simulink model "generate_cartesian_pose_motion"  (R2023a)
settings: Solver=FixedStepDiscrete  StartTime=0.0  StopTime=inf  FixedStep=0.001  RelTol=1e-3  EnableMultiTasking=on
PreLoadFcn:
  | frs = FrankaRobotSettings;
libraries: franka_simulink_library x4
settings Model: SimulationMode=external  ExtModeTrigDuration=10000  Creator=vasi_ko  LastModifiedBy=kvasios
settings SolverCC: AlgebraicLoopSolver=TrustRegion
settings DataIOCC: LimitDataPoints=on  SaveFormat=Array  ReturnWorkspaceOutputs=off
settings OptimizationCC: DefaultParameterBehavior=Inlined  EnhancedBackFolding=on  PassReuseOutputArgsThreshold=0  OptimizeBlockOrder=speed  DifferentSizesBufferReuse=on  OptimizationCustomize=off
settings DebuggingCC: SolverPrmCheckMsg=warning  ParameterTunabilityLossMsg=error  UnconnectedInputMsg=warning  UnconnectedOutputMsg=warning  UnconnectedLineMsg=warning  SFUnexpectedBacktrackingDiag=warning  SFNoUnconditionalDefaultTransitionDiag=warning  SFExecutionAtInitializationDiag=none  ArithmeticOperatorsInVariantConditions=warning
settings ModelReferenceCC: EnableRefExpFcnMdlSchedulingChecks=on  PropagateSignalLabelsOutOfModel=off
settings SFSimCC: SimUseLocalCustomCode=off  MATLABDynamicMemAlloc=off  CustomCodeUndefinedFunction=UseInterfaceOnly  SimTargetLang=C++
settings RTWCC: RTWVerbose=off  RTWUseLocalCustomCode=off  BuildConfiguration=Faster Runs  TargetLang=C++  DLArmComputeVersion=19.05
settings CodeAppCC: ForceParamTrailComments=on  OperatorAnnotations=on
settings ConfigComp: CovMetricSettings=dw  CovSaveCumulativeToWorkspaceVar=on  CovSaveSingleToWorkspaceVar=on  CovExternalEMLEnable=off  CovSFcnEnable=off

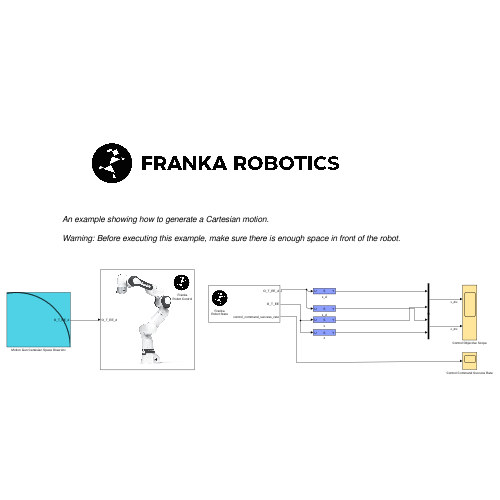
[thumbnail: Simulink's stored preview of the top-level diagram]
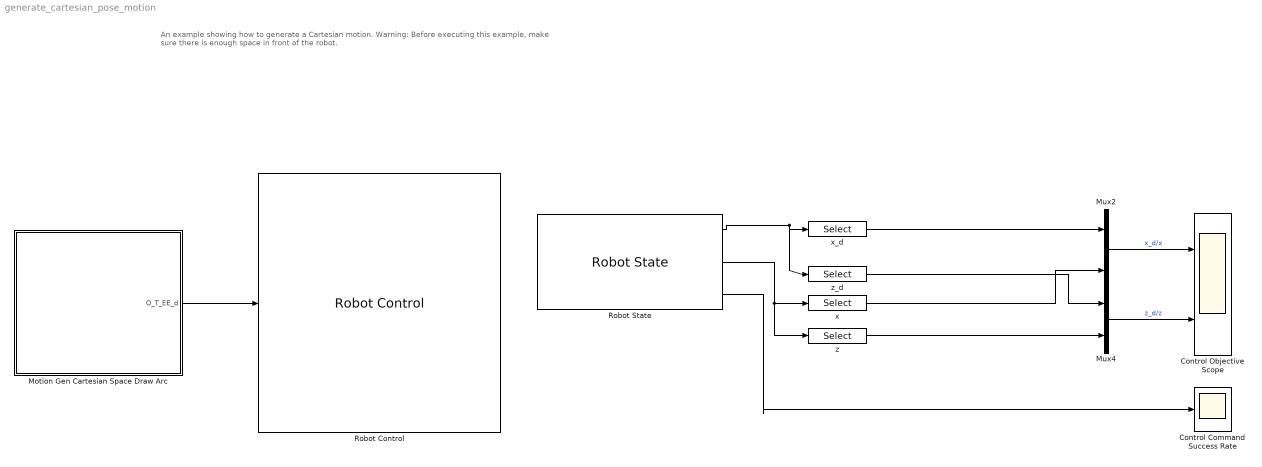
== system generate_cartesian_pose_motion ==
  note: An example showing how to generate a Cartesian motion.
      |
      | Warning: Before executing this example, make sure there is enough space in front of the robot.
  Control Command Success Rate : Scope
  Control Objective Scope : Scope  NumInputPorts=2
  Motion Gen Cartesian Space Draw Arc : Subsystem
      mask Display:
      | pos = get_param(gcb, 'Position');
      | width = pos(3) - pos(1);
      | x = [0:width];
      | y = sin(x/180*pi);
      | % Parameters 'm' and 'b' must be defined in 'Parameters & Dialog' pane.
      | plot(cos(x/180*pi*0.5), sin(x/180*pi*0.5));
      | 
      | port_label('output',1,'O_T_EE_d');
  Mux2 : Mux  Inputs=2
  Mux4 : Mux  Inputs=2
  Robot Control : franka_simulink_library/Robot Control  robot_ip=frs.robot_ip  gripper_selection=None  control_mode=Cartesian Pose - Internal Controller Mode  controller_choice=Joint Impedance Controller  joint_impedance=frs.joint_impedance_stiffness  cartesian_impedance=[3000, 3000, 3000, 300, 300, 300]  rate_limiter=on  cuttoff_frequency=frs.cutoff_frequency  elbow_control=off  collision_thresholds=frs.collision_thresholds.getAs1DArray  load_inertia=frs.load_inertia.getAs1DArray  NE_T_EE=frs.NE_T_EE(:)  EE_T_K=frs.EE_T_K(:)  init_joint_configuration_req=on  init_joint_configuration=frs.home_configuration
      settings: SourceProductName=Franka Robotics Simulink Support Package
  Robot State : franka_simulink_library/Robot State  robot_ip=frs.robot_ip  signals_requested='O_T_EE_d O_T_EE control_command_success_rate'
      settings: SourceProductName=Franka Robotics Simulink Support Package
  x : Selector  InputPortWidth=16  IndexOptions=Index vector (dialog)  Indices=13  OutputSizes=1
  x_d : Selector  InputPortWidth=16  IndexOptions=Index vector (dialog)  Indices=13  OutputSizes=1
  z : Selector  InputPortWidth=16  IndexOptions=Index vector (dialog)  Indices=15  OutputSizes=1
  z_d : Selector  InputPortWidth=16  IndexOptions=Index vector (dialog)  Indices=15  OutputSizes=1
  wires:
  x/1 -> Mux2/2
  z/1 -> Mux4/2
  Mux2/1 -> Control Objective Scope/1  "x_d/x"
  Mux4/1 -> Control Objective Scope/2  "z_d/z"
  Robot State/1 -> z_d/1, x_d/1
  x_d/1 -> Mux2/1
  Motion Gen Cartesian Space Draw Arc/1(O_T_EE_d) -> Robot Control/1
  z_d/1 -> Mux4/1
  Robot State/2 -> z/1, x/1
  Robot State/3 -> Control Command Success Rate/1

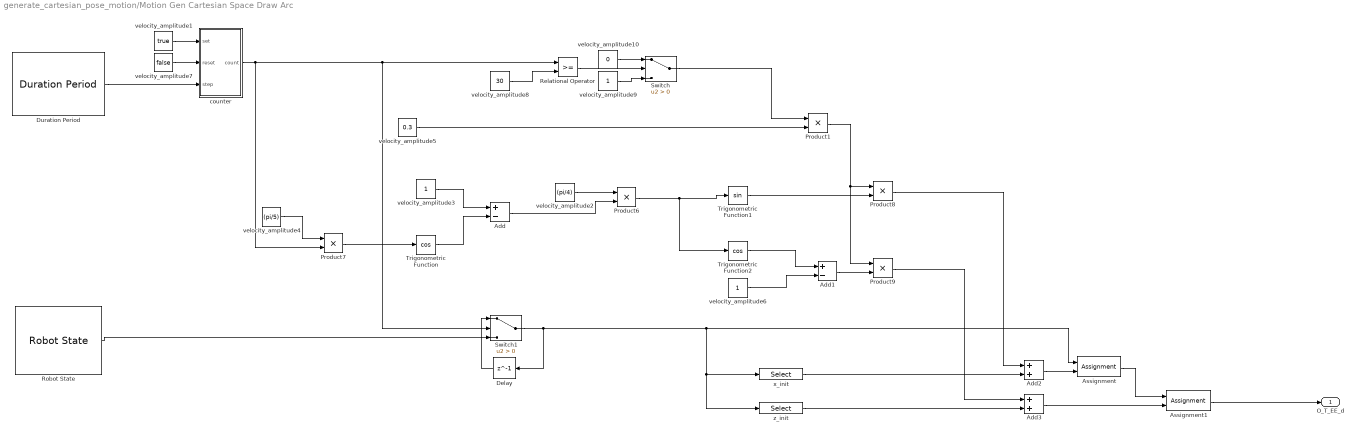
== system generate_cartesian_pose_motion/Motion Gen Cartesian Space Draw Arc ==
  Add : Sum  Inputs=+-
  Add1 : Sum  Inputs=+-
  Add2 : Sum
  Add3 : Sum
  Assignment : Assignment  DiagnosticForDimensions=Warning  IndexOptions=Index vector (dialog)  Indices=13  OutputSizes=1
  Assignment1 : Assignment  DiagnosticForDimensions=Warning  IndexOptions=Index vector (dialog)  Indices=15  OutputSizes=1
  Delay : Delay  DelayLength=1
  Duration Period : franka_simulink_library/Duration Period  robot_ip=frs.robot_ip
      settings: SourceProductName=Franka Robotics Simulink Support Package
  Product{1,6..9} (5 alike) : Product
  Relational Operator : RelationalOperator  OutDataTypeStr=boolean  InputSameDT=off
  Robot State : franka_simulink_library/Robot State  robot_ip=frs.robot_ip  signals_requested='O_T_EE_c'
      settings: SourceProductName=Franka Robotics Simulink Support Package
  Switch : Switch  Criteria=u2 > Threshold  SaturateOnIntegerOverflow=off  InputSameDT=off
  Switch1 : Switch  Criteria=u2 > Threshold  SaturateOnIntegerOverflow=off  InputSameDT=off
  Trigonometric Function : Trigonometry  Operator=cos  NumberOfIterations=50
  Trigonometric Function1 : Trigonometry  NumberOfIterations=50
  Trigonometric Function2 : Trigonometry  Operator=cos
  counter : Subsystem
  velocity_amplitude1 : Constant  Value=true  VectorParams1D=off
  velocity_amplitude10 : Constant  Value=0  VectorParams1D=off
  velocity_amplitude2 : Constant  Value=(pi/4)  VectorParams1D=off
  velocity_amplitude3 : Constant  VectorParams1D=off
  velocity_amplitude4 : Constant  Value=(pi/5)  VectorParams1D=off
  velocity_amplitude5 : Constant  Value=0.3  VectorParams1D=off
  velocity_amplitude6 : Constant  VectorParams1D=off
  velocity_amplitude7 : Constant  Value=false  VectorParams1D=off
  velocity_amplitude8 : Constant  Value=30  VectorParams1D=off
  velocity_amplitude9 : Constant  VectorParams1D=off
  x_init : Selector  InputPortWidth=16  IndexOptions=Index vector (dialog)  Indices=13  OutputSizes=1
  z_init : Selector  InputPortWidth=16  IndexOptions=Index vector (dialog)  Indices=15  OutputSizes=1
  O_T_EE_d : Outport  VectorParamsAs1DForOutWhenUnconnected=off
  wires:
  Product8/1 -> Add2/1
  x_init/1 -> Add2/2
  Assignment/1 -> Assignment1/1
  Add2/1 -> Assignment/2
  Switch1/1 -> Delay/1, z_init/1, x_init/1, Assignment/1
  velocity_amplitude2/1 -> Product6/1
  velocity_amplitude3/1 -> Add/1
  velocity_amplitude4/1 -> Product7/1
  Trigonometric Function/1 -> Add/2
  Product7/1 -> Trigonometric Function/1
  Add/1 -> Product6/2
  Product6/1 -> Trigonometric Function1/1, Trigonometric Function2/1
  Trigonometric Function1/1 -> Product8/2
  Trigonometric Function2/1 -> Add1/1
  velocity_amplitude6/1 -> Add1/2
  Add1/1 -> Product9/2
  velocity_amplitude5/1 -> Product1/2
  Switch/1 -> Product1/1
  Product1/1 -> Product9/1, Product8/1
  Add3/1 -> Assignment1/2
  Duration Period/1 -> counter/3(step)
  velocity_amplitude1/1 -> counter/1(set)
  velocity_amplitude7/1 -> counter/2(reset)
  counter/1(count) -> Product7/2, Relational Operator/1, Switch1/2
  Assignment1/1 -> O_T_EE_d/1
  z_init/1 -> Add3/2
  Product9/1 -> Add3/1
  velocity_amplitude8/1 -> Relational Operator/2
  Relational Operator/1 -> Switch/2
  velocity_amplitude9/1 -> Switch/3
  velocity_amplitude10/1 -> Switch/1
  Delay/1 -> Switch1/1
  Robot State/1 -> Switch1/3

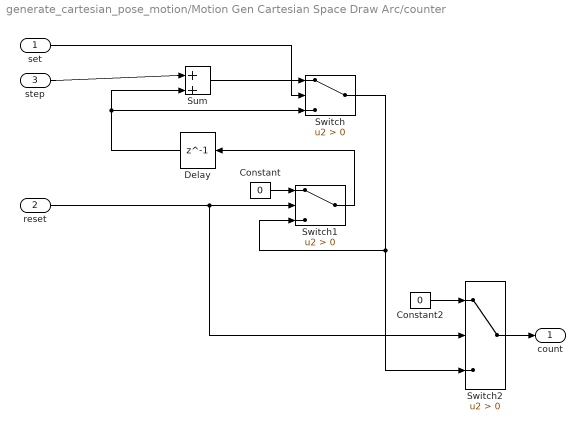
== system generate_cartesian_pose_motion/Motion Gen Cartesian Space Draw Arc/counter ==
  set : Inport  OutDataTypeStr=boolean
  reset : Inport  Port=2  OutDataTypeStr=boolean
  step : Inport  Port=3  OutDataTypeStr=double
  Constant : Constant  Value=0  OutDataTypeStr=double
  Constant2 : Constant  Value=0  OutDataTypeStr=double
  Delay : Delay  DelayLength=1  InitialCondition=0
  Sum : Sum  Inputs=|++
  Switch : Switch  Criteria=u2 > Threshold  SaturateOnIntegerOverflow=off  InputSameDT=off
  Switch1 : Switch  Criteria=u2 > Threshold  OutDataTypeStr=double  SaturateOnIntegerOverflow=off  InputSameDT=off
  Switch2 : Switch  Criteria=u2 > Threshold  OutDataTypeStr=double  SaturateOnIntegerOverflow=off  InputSameDT=off
  count : Outport  OutDataTypeStr=double  VectorParamsAs1DForOutWhenUnconnected=off
  wires:
  Switch1/1 -> Delay/1
  Constant/1 -> Switch1/1
  reset/1 -> Switch2/2, Switch1/2
  Delay/1 -> Switch/3, Sum/2
  step/1 -> Sum/1
  Switch/1 -> Switch2/3, Switch1/3
  set/1 -> Switch/2
  Sum/1 -> Switch/1
  Constant2/1 -> Switch2/1
  Switch2/1 -> count/1
